simulink model "reaction_wheel"  (R2023b)
settings: Solver=ode3  StartTime=0.0  StopTime=200  FixedStep=0.1  RelTol=1e-3
values from neighbouring files (symbols this model uses):
  A = [-a a a -a; -a -a a a; a a a a]    [reaction_wheels.m]    (also in reaction_wheels_code.m = eye(3))
  A_ = [-b -b b; b -b b; b b b; -b b b]    [reaction_wheels.m]    (also in reaction_wheels_code.m)
  h_r_0 = [0 0 0 0]'    [reaction_wheels.m]    (also in reaction_wheels_code.m = [0 0 0]')
  I = [Ix 0 0; 0 Iy 0; 0 0 Iz]    [reaction_wheels.m]    (also in reaction_wheels_code.m)
  I_inv = inv(I)    [reaction_wheels.m]    (also in reaction_wheels_code.m)
  M = 0    [reaction_wheels.m]    (also in reaction_wheels_code.m)
  M_c = [1 0 0]'    [reaction_wheels.m]    (also in reaction_wheels_code.m)
  omega_0 = [0 0 0]'    [reaction_wheels.m]    (also in reaction_wheels_code.m)
libraries: matrix_library x2
settings Model: Creator=valen  LastModifiedBy=valen

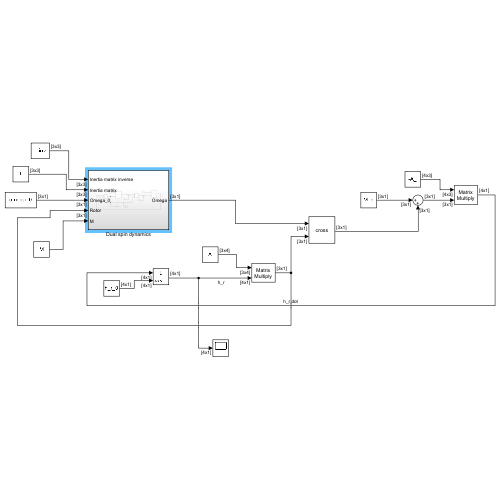
[thumbnail: Simulink's stored preview of the top-level diagram]
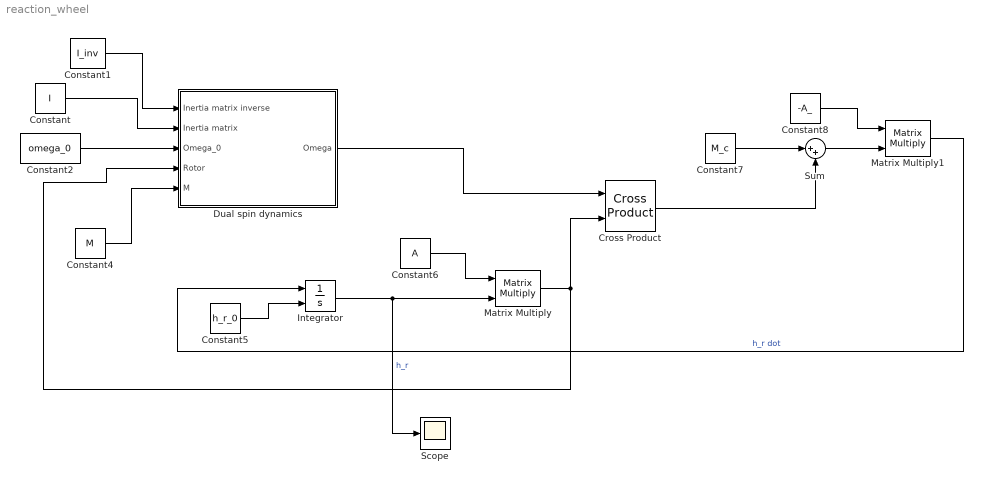
== system reaction_wheel ==
  Constant : Constant  Value=I  VectorParams1D=off
  Constant1 : Constant  Value=I_inv  VectorParams1D=off
  Constant2 : Constant  Value=omega_0  VectorParams1D=off
  Constant4 : Constant  Value=M  VectorParams1D=off
  Constant5 : Constant  Value=h_r_0  VectorParams1D=off
  Constant6 : Constant  Value=A  VectorParams1D=off
  Constant7 : Constant  Value=M_c  VectorParams1D=off
  Constant8 : Constant  Value=-A_  VectorParams1D=off
  Cross Product : matrix_library/Cross Product
  Dual spin dynamics : Subsystem
  Integrator : Integrator  InitialConditionSource=external
  Matrix Multiply : Product  Multiplication=Matrix(*)
  Matrix Multiply1 : Product  Multiplication=Matrix(*)
  Scope : Scope
  Sum : Sum  Inputs=|++
  wires:
  Constant1/1 -> Dual spin dynamics/1(Inertia matrix inverse)
  Constant/1 -> Dual spin dynamics/2(Inertia matrix)
  Constant2/1 -> Dual spin dynamics/3(Omega_0)
  Matrix Multiply/1 -> Cross Product/2, Dual spin dynamics/4(Rotor)
  Constant4/1 -> Dual spin dynamics/5(M)
  Constant5/1 -> Integrator/2
  Integrator/1 -> Scope/1, Matrix Multiply/2  "h_r"
  Constant6/1 -> Matrix Multiply/1
  Dual spin dynamics/1(Omega) -> Cross Product/1
  Cross Product/1 -> Sum/2
  Constant7/1 -> Sum/1
  Sum/1 -> Matrix Multiply1/2
  Constant8/1 -> Matrix Multiply1/1
  Matrix Multiply1/1 -> Integrator/1  "h_r dot"

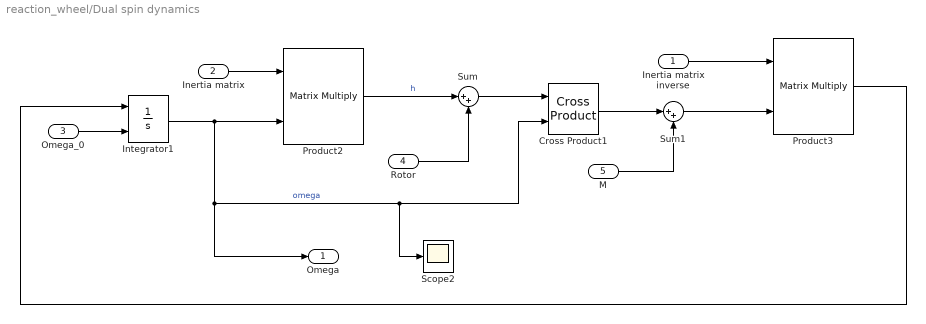
== system reaction_wheel/Dual spin dynamics ==
  Inertia matrix inverse : Inport
  Inertia matrix : Inport  Port=2
  Omega_0 : Inport  Port=3
  Rotor : Inport  Port=4
  M : Inport  Port=5
  Cross Product1 : matrix_library/Cross Product
  Integrator1 : Integrator  InitialConditionSource=external
  Product2 : Product  Multiplication=Matrix(*)
  Product3 : Product  Multiplication=Matrix(*)
  Scope2 : Scope
  Sum : Sum  Inputs=|++
  Sum1 : Sum  Inputs=|++
  Omega : Outport
  wires:
  M/1 -> Sum1/2
  Sum1/1 -> Product3/2
  Omega_0/1 -> Integrator1/2
  Product2/1 -> Sum/1  "h"
  Inertia matrix/1 -> Product2/1
  Product3/1 -> Integrator1/1
  Rotor/1 -> Sum/2
  Integrator1/1 -> Product2/2, Omega/1, Scope2/1, Cross Product1/2  "omega"
  Cross Product1/1 -> Sum1/1
  Inertia matrix inverse/1 -> Product3/1
  Sum/1 -> Cross Product1/1
